simulink model "PCIe_UserLogic_00"  (Simulink 7.6)
settings: Solver=ode45  StartTime=0.0  StopTime=10.0  RelTol=1e-3
PreLoadFcn:
  | SP605_TS  = 1/200e6;
  | SP605_CLK = SP605_TS*1e9;
  | USER_TS  = 1/200e6;
  | USER_CLK = USER_TS*1e9;
  | 
  | PCIE_TS   = 1/125e6;
  | PCIE_CLK = PCIE_TS*1e9;
  | 
  | P_Size = 32;
  | 
  | WR_LAT = 10 + round(P_Size*5/12);
InitFcn:
  | SP605_TS  = 1/200e6;
  | SP605_CLK = SP605_TS*1e9;
  | USER_TS  = 1/200e6;
  | USER_CLK = USER_TS*1e9;
  | 
  | PCIE_TS   = 1/125e6;
  | PCIE_CLK = PCIE_TS*1e9;
  | 
  | P_Size = 32;
  | 
  | WR_LAT = 10 + round(P_Size*5/12);
libraries: xbsIndex_r4 x341
(part 1 of 3)
CloseFcn:
  | rtwprivate ssgencode ModelCloseRequest MIG_Test_01
settings Model: Creator=Gigi  LastModifiedBy=root

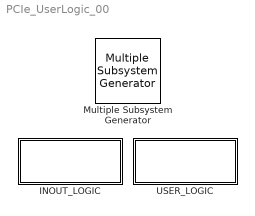
== system PCIe_UserLogic_00 ==
  INOUT_LOGIC : Subsystem
  Multiple Subsystem Generator : xbsIndex_r4/Multiple Subsystem Generator  Tag=xlStitcher  block_type=multiple_subsystem_generator
      settings: infoedit=Multiple Subsystem\nGenerator  block_version=12.3
  USER_LOGIC : Subsystem
